simulink model "cc_aqm_delay"  (R2014a)
settings: Solver=ode45  StartTime=0.0  StopTime=10.0  RelTol=1e-3
undefined symbols (not defined in the file): C, MSR_US, N, q_ref, R0
libraries: simulink x2
settings Model: Creator=tohoanglinh  LastModifiedBy=linhth
settings DebuggingCC: UnderspecifiedInitializationDetection=Classic  StateNameClashWarn=warning

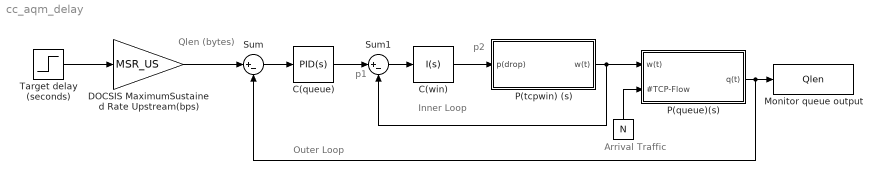
== system cc_aqm_delay ==
  note: Arrival Traffic
  note: Qlen (bytes)
  note: p2
  note: Outer Loop
  note: p1
  note: Inner Loop
  " " : Constant  Value=N
  C(queue) : simulink/Continuous/PID Controller  Controller=PID  TimeDomain=Continuous-time  SampleTime=1  IntegratorMethod=Forward Euler  FilterMethod=Forward Euler  Form=Parallel  P=1  I=1  D=0  N=100  InitialConditionSource=internal  InitialConditionForIntegrator=0  InitialConditionForFilter=0  ExternalReset=none  LimitOutput=off  UpperSaturationLimit=inf  LowerSaturationLimit=-inf  LinearizeAsGain=on  AntiWindupMode=none  Kb=1  TrackingMode=off  Kt=1  PParamMin=[]  PParamMax=[]  IParamMin=[]  IParamMax=[]  DParamMin=[]  DParamMax=[]  NParamMin=[]  NParamMax=[]  KbParamMin=[]  KbParamMax=[]  KtParamMin=[]  KtParamMax=[]  POutMin=[]  POutMax=[]  IOutMin=[]  IOutMax=[]  DOutMin=[]  DOutMax=[]  NOutMin=[]  NOutMax=[]  KbOutMin=[]  KbOutMax=[]  KtOutMin=[]  KtOutMax=[]  IntegratorOutMin=[]  IntegratorOutMax=[]  FilterOutMin=[]  FilterOutMax=[]  SumOutMin=[]  SumOutMax=[]  SumI1OutMin=[]  SumI1OutMax=[]  SumI2OutMin=[]  SumI2OutMax=[]  SumI3OutMin=[]  SumI3OutMax=[]  SumDOutMin=[]  SumDOutMax=[]  SaturationOutMin=[]  SaturationOutMax=[]  IntegratorContinuousStateAttributes=''  IntegratorStateMustResolveToSignalObject=off  IntegratorRTWStateStorageClass=Auto  FilterContinuousStateAttributes=''  FilterStateMustResolveToSignalObject=off  FilterRTWStateStorageClass=Auto
  C(win) : simulink/Continuous/PID Controller  Controller=I  TimeDomain=Continuous-time  SampleTime=1  IntegratorMethod=Forward Euler  FilterMethod=Forward Euler  Form=Parallel  P=1  I=1  D=0  N=100  InitialConditionSource=internal  InitialConditionForIntegrator=0  InitialConditionForFilter=0  ExternalReset=none  LimitOutput=off  UpperSaturationLimit=inf  LowerSaturationLimit=-inf  LinearizeAsGain=on  AntiWindupMode=none  Kb=1  TrackingMode=off  Kt=1  PParamMin=[]  PParamMax=[]  IParamMin=[]  IParamMax=[]  DParamMin=[]  DParamMax=[]  NParamMin=[]  NParamMax=[]  KbParamMin=[]  KbParamMax=[]  KtParamMin=[]  KtParamMax=[]  POutMin=[]  POutMax=[]  IOutMin=[]  IOutMax=[]  DOutMin=[]  DOutMax=[]  NOutMin=[]  NOutMax=[]  KbOutMin=[]  KbOutMax=[]  KtOutMin=[]  KtOutMax=[]  IntegratorOutMin=[]  IntegratorOutMax=[]  FilterOutMin=[]  FilterOutMax=[]  SumOutMin=[]  SumOutMax=[]  SumI1OutMin=[]  SumI1OutMax=[]  SumI2OutMin=[]  SumI2OutMax=[]  SumI3OutMin=[]  SumI3OutMax=[]  SumDOutMin=[]  SumDOutMax=[]  SaturationOutMin=[]  SaturationOutMax=[]  IntegratorContinuousStateAttributes=''  IntegratorStateMustResolveToSignalObject=off  IntegratorRTWStateStorageClass=Auto  FilterContinuousStateAttributes=''  FilterStateMustResolveToSignalObject=off  FilterRTWStateStorageClass=Auto
  DOCSIS MaximumSustained Rate Upstream(bps) : Gain  Gain=MSR_US
  Monitor queue output : ToWorkspace  VariableName=Qlen  SaveFormat=Timeseries  SampleTime=-1
  P(queue)(s) : Subsystem
  P(tcpwin) (s) : Subsystem
  Sum : Sum  Inputs=|+-
  Sum1 : Sum  Inputs=|+-
  Target delay (seconds) : Step  Time=q_ref  SampleTime=0
  wires:
  P(tcpwin) (s)/1(w(t)) -> P(queue)(s)/1(w(t)), Sum1/2
  P(queue)(s)/1(q(t)) -> Monitor queue output/1, Sum/2
  C(win)/1 -> P(tcpwin) (s)/1(p(drop))
  C(queue)/1 -> Sum1/1
  DOCSIS MaximumSustained Rate Upstream(bps)/1 -> Sum/1
  " "/1 -> P(queue)(s)/2(#TCP-Flow)
  Sum/1 -> C(queue)/1
  Sum1/1 -> C(win)/1
  Target delay (seconds)/1 -> DOCSIS MaximumSustained Rate Upstream(bps)/1

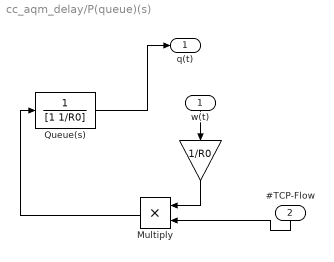
== system cc_aqm_delay/P(queue)(s) ==
  w(t) : Inport
  #TCP-Flow : Inport  Port=2
  " " : Gain  Gain=1/R0
  Multiply : Product
  Queue(s) : TransferFcn  Denominator=[1 1/R0]
  q(t) : Outport
  wires:
  Queue(s)/1 -> q(t)/1
  " "/1 -> Multiply/1
  w(t)/1 -> " "/1
  #TCP-Flow/1 -> Multiply/2
  Multiply/1 -> Queue(s)/1

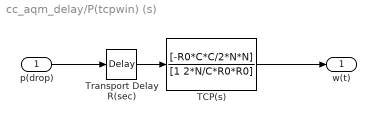
== system cc_aqm_delay/P(tcpwin) (s) ==
  p(drop) : Inport
  TCP(s) : TransferFcn  Numerator=[-R0*C*C/2*N*N]  Denominator=[1 2*N/C*R0*R0]
  Transport Delay R(sec) : TransportDelay
  w(t) : Outport
  wires:
  Transport Delay R(sec)/1 -> TCP(s)/1
  p(drop)/1 -> Transport Delay R(sec)/1
  TCP(s)/1 -> w(t)/1
